simulink model "verify_Inverter_CONF_mdl"  (R2016b)
settings: Solver=ode45  StartTime=0.0  StopTime=15  MaxStep=1  RelTol=1e-3  EnableMultiTasking=on
undefined symbols (not defined in the file or in its folder): path_carnot
libraries: carnot x3, simulink x1
settings Model: Creator=drhf  LastModifiedBy=drhf
settings DataIOCC: SaveFormat=Array  SignalLoggingSaveFormat=ModelDataLogs
settings OptimizationCC: ExpressionDepthLimit=2147483647  LifeSpan=inf
settings DebuggingCC: UnderspecifiedInitializationDetection=Classic  MergeDetectMultiDrivingBlocksExec=none  SolverPrmCheckMsg=warning  FcnCallInpInsideContextMsg=warning  StateNameClashWarn=warning  SFUnexpectedBacktrackingDiag=warning  SFNoUnconditionalDefaultTransitionDiag=warning  SFExecutionAtInitializationDiag=none
settings HardwareCC: ProdBitPerPointer=32  ProdBitPerSizeT=32  ProdBitPerPtrDiffT=32  ProdLargestAtomicFloat=None  ProdIntDivRoundTo=Undefined  ProdEndianess=Unspecified  ProdWordSize=32  ProdHWDeviceType=32-bit Generic
settings ModelReferenceCC: PropagateSignalLabelsOutOfModel=off
settings GRTTargetCC: TargetLangStandard=C89/C90 (ANSI)  GeneratePreprocessorConditionals=Disable all  CombineOutputUpdateFcns=off  GRTInterface=on
settings ConfigComp: CovMetricSettings=dw  CovHtmlReporting=on  CovSaveCumulativeToWorkspaceVar=on  CovSaveSingleToWorkspaceVar=on  CovExternalEMLEnable=off

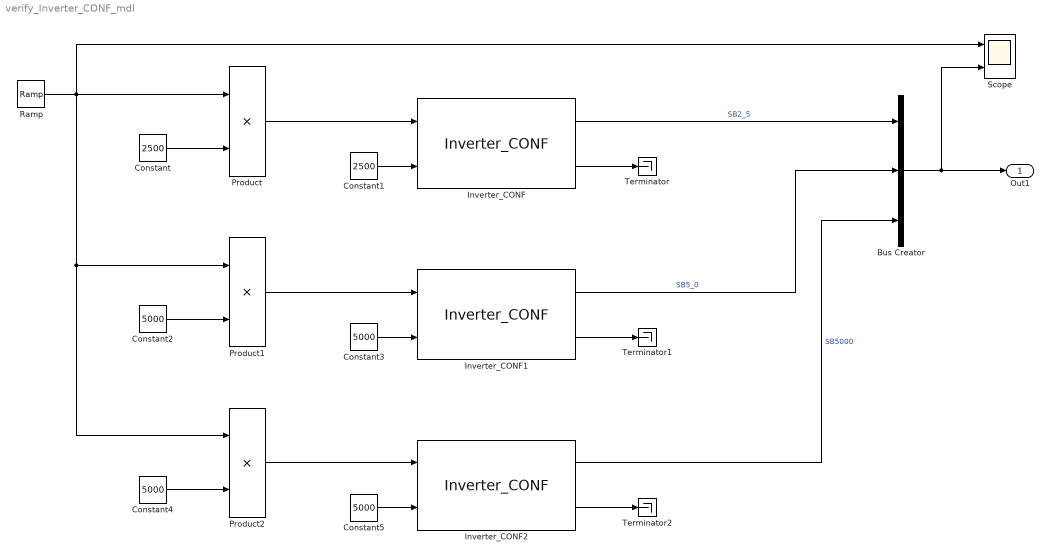
== system verify_Inverter_CONF_mdl ==
  Bus Creator : BusCreator  Inputs=3
  Constant : Constant  Value=2500
  Constant1 : Constant  Value=2500
  Constant{2..5} (4 alike) : Constant  Value=5000
  Inverter_CONF : carnot/Source/Electric_Generator/Inverter_CONF  PathName=fullfile(path_carnot('libsl'), 'Source','Electric_Generator','Inverter_CONF','parameter_set')  FileName='SMA_SB2_5_VL40.mat'  userPath=off  userParam=off  Pacnom=2500  overload=1  PstepsEta=[0 0.1 0.2 0.25 0.3 0.5 0.75 1]  Eta=[0 0.948 0.966 0.969 0.97 0.972 0.97 0.967]  P_standby=2
  Inverter_CONF1 : carnot/Source/Electric_Generator/Inverter_CONF  PathName=fullfile(path_carnot('libsl'), 'Source','Electric_Generator','Inverter_CONF','parameter_set')  FileName='SMA_SB5_0_AV40.mat'  userPath=off  userParam=off  Pacnom=5000  overload=1  PstepsEta=[0 0.1 0.2 0.25 0.3 0.5 0.75 1]  Eta=[0 0.952 0.966 0.968 0.97 0.97 0.967 0.962]  P_standby=1
  Inverter_CONF2 : carnot/Source/Electric_Generator/Inverter_CONF  PathName=fullfile(path_carnot('libsl'), 'Source','Electric_Generator','Inverter_CONF','parameter_set')  FileName='SMA_SB5000_TL21.mat'  userPath=off  userParam=off  Pacnom=5000  overload=1  PstepsEta=[0 0.1 0.2 0.25 0.3 0.5 0.75 1]  Eta=[0 0.944 0.961 0.964 0.967 0.97 0.971 0.97]  P_standby=1
  Product : Product
  Product1 : Product
  Product2 : Product
  Ramp : simulink/Sources/Ramp  slope=0.1  start=0  X0=0
  Scope : Scope  NumInputPorts=2
  Terminator : Terminator
  Terminator1 : Terminator
  Terminator2 : Terminator
  Out1 : Outport
  wires:
  Constant/1 -> Product/2
  Product/1 -> Inverter_CONF/1
  Constant1/1 -> Inverter_CONF/2
  Inverter_CONF/2 -> Terminator/1
  Inverter_CONF/1 -> Bus Creator/1  "SB2_5"
  Constant2/1 -> Product1/2
  Product1/1 -> Inverter_CONF1/1
  Constant3/1 -> Inverter_CONF1/2
  Inverter_CONF1/2 -> Terminator1/1
  Inverter_CONF1/1 -> Bus Creator/2  "SB5_0"
  Ramp/1 -> Scope/1, Product2/1, Product1/1, Product/1
  Constant4/1 -> Product2/2
  Product2/1 -> Inverter_CONF2/1
  Constant5/1 -> Inverter_CONF2/2
  Inverter_CONF2/2 -> Terminator2/1
  Inverter_CONF2/1 -> Bus Creator/3  "SB5000"
  Bus Creator/1 -> Scope/2, Out1/1
